simulink model "tiltrotor_model5"  (R2023a)
settings: Solver=FixedStepAuto  StartTime=0.0  StopTime=30  FixedStep=1e-3  RelTol=1e-3
values from neighbouring files (symbols this model uses):
  g = 9.81    [LQR_controller_pitching.m]    (also in MPC_controller_pitching.m; MPC_vs_LQR.m; simulation_parameters.m)
  I = diag([0.018 0.035 0.051])    [simulation_parameters.m]
  initial = [0 0 0 0 0 0]'    [simulation_parameters.m]
  kf = 65    [simulation_parameters.m]
  Lh = 0.2    [simulation_parameters.m]
  Lv = 0.2    [simulation_parameters.m]
  m = 1.12    [LQR_controller_pitching.m]    (also in MPC_vs_LQR.m = size(Bd,2); simulation_parameters.m)
  p_D = 0    [controller_parameters_model_5_and_6.m]
  p_I = 0    [controller_parameters_model_5_and_6.m]
  p_P = 0.35    [controller_parameters_model_5_and_6.m]
  pitch_D = 0.4    [controller_parameters.m]    (also in controller_parameters_model_3_and_4.m; controller_parameters_model_5_and_6.m = 0)
  pitch_I = 0    [controller_parameters.m]    (also in controller_parameters_model_3_and_4.m; controller_parameters_model_5_and_6.m)
  pitch_P = 1.4    [controller_parameters.m]    (also in controller_parameters_model_3_and_4.m; controller_parameters_model_5_and_6.m = 10)
  r_D = 0    [controller_parameters_model_5_and_6.m]
  r_I = 0    [controller_parameters_model_5_and_6.m]
  r_P = 1    [controller_parameters_model_5_and_6.m]
  reference = [1 1 1 0 40 50]'    [simulation_parameters.m]
  roll_D = 0.3    [controller_parameters.m]    (also in controller_parameters_model_3_and_4.m; controller_parameters_model_5_and_6.m = 1)
  roll_I = 0    [controller_parameters.m]    (also in controller_parameters_model_3_and_4.m; controller_parameters_model_5_and_6.m)
  roll_P = 1.5    [controller_parameters.m]    (also in controller_parameters_model_3_and_4.m; controller_parameters_model_5_and_6.m = 8)
  s_r = [1 1 1 1 1 1]    [simulation_parameters.m]
  Tmax = 4    [simulation_parameters.m]
  toll = 1e-12    [simulation_parameters.m]
  vy_D = 0    [controller_parameters.m]    (also in controller_parameters_model_3_and_4.m; controller_parameters_model_5_and_6.m)
  vy_I = 0    [controller_parameters.m]    (also in controller_parameters_model_3_and_4.m; controller_parameters_model_5_and_6.m)
  vy_P = 5    [controller_parameters.m]    (also in controller_parameters_model_3_and_4.m; controller_parameters_model_5_and_6.m = 12)
  x_D = 0.7    [controller_parameters.m]    (also in controller_parameters_model_3_and_4.m; controller_parameters_model_5_and_6.m = 0)
  x_I = 0    [controller_parameters.m]    (also in controller_parameters_model_3_and_4.m; controller_parameters_model_5_and_6.m)
  x_P = 1.8    [controller_parameters.m]    (also in controller_parameters_model_3_and_4.m; controller_parameters_model_5_and_6.m = 1.5)
  y_D = 0.7    [controller_parameters.m]    (also in controller_parameters_model_3_and_4.m; controller_parameters_model_5_and_6.m = 0.3)
  y_I = 0    [controller_parameters.m]    (also in controller_parameters_model_3_and_4.m; controller_parameters_model_5_and_6.m)
  y_P = 1.8    [controller_parameters.m]    (also in controller_parameters_model_3_and_4.m; controller_parameters_model_5_and_6.m = 1.5)
  yaw_D = 0.5    [controller_parameters.m]    (also in controller_parameters_model_3_and_4.m = 0.3; controller_parameters_model_5_and_6.m = 0)
  yaw_I = 0    [controller_parameters.m]    (also in controller_parameters_model_3_and_4.m; controller_parameters_model_5_and_6.m)
  yaw_P = 1    [controller_parameters.m]    (also in controller_parameters_model_3_and_4.m; controller_parameters_model_5_and_6.m = 1.5)
  z_D = 0    [controller_parameters.m]    (also in controller_parameters_model_3_and_4.m; controller_parameters_model_5_and_6.m)
  z_I = 0    [controller_parameters.m]    (also in controller_parameters_model_3_and_4.m; controller_parameters_model_5_and_6.m)
  z_P = 3    [controller_parameters.m]    (also in controller_parameters_model_3_and_4.m; controller_parameters_model_5_and_6.m = 2.5)
undefined symbols (not defined in the file or in its folder): K
libraries: slpidlib x9, simulink x6, simulink_extras x1, matrix_library x1
(part 1 of 2)
settings Model: Creator=and20  LastModifiedBy=and20

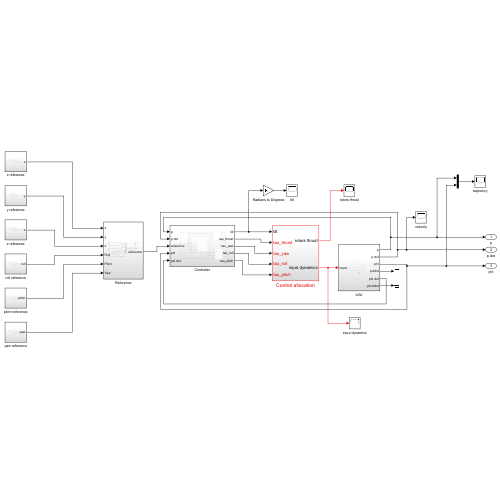
[thumbnail: Simulink's stored preview of the top-level diagram]
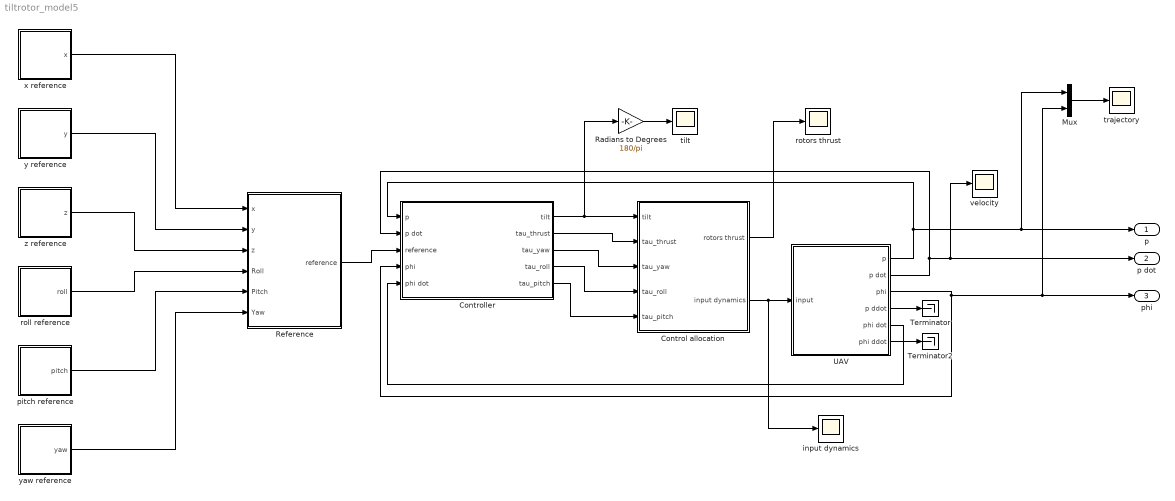
== system tiltrotor_model5 ==
  Control allocation : Subsystem
  Controller : Subsystem
  Mux : Mux  Inputs=2
  Radians to Degrees : Gain  Gain=180/pi
  Reference : Subsystem
  Terminator : Terminator
  Terminator2 : Terminator
  UAV : Subsystem
  input dynamics : Scope
  pitch reference : Subsystem
  roll reference : Subsystem
  rotors thrust : Scope
  tilt : Scope
  trajectory : Scope
  velocity : Scope
  x reference : Subsystem
  y reference : Subsystem
  yaw reference : Subsystem
  z reference : Subsystem
  p : Outport
  p dot : Outport  Port=2
  phi : Outport  Port=3
  wires:
  Reference/1(reference) -> Controller/3(reference)
  UAV/2(p dot) -> Controller/2(p dot), velocity/1, p dot/1
  UAV/3(phi) -> Mux/2, phi/1, Controller/4(phi)
  Mux/1 -> trajectory/1
  UAV/1(p) -> Controller/1(p), Mux/1, p/1
  x reference/1(x) -> Reference/1(x)
  y reference/1(y) -> Reference/2(y)
  z reference/1(z) -> Reference/3(z)
  roll reference/1(roll) -> Reference/4(Roll)
  pitch reference/1(pitch) -> Reference/5(Pitch)
  yaw reference/1(yaw) -> Reference/6(Yaw)
  Radians to Degrees/1 -> tilt/1
  UAV/4(p ddot) -> Terminator/1
  UAV/5(phi dot) -> Controller/5(phi dot)
  UAV/6(phi ddot) -> Terminator2/1
  Controller/1(tilt) -> Radians to Degrees/1, Control allocation/1(tilt)
  Controller/2(tau_thrust) -> Control allocation/2(tau_thrust)
  Controller/3(tau_yaw) -> Control allocation/3(tau_yaw)
  Controller/4(tau_roll) -> Control allocation/4(tau_roll)
  Controller/5(tau_pitch) -> Control allocation/5(tau_pitch)
  Control allocation/2(input dynamics) -> input dynamics/1, UAV/1(input)
  Control allocation/1(rotors thrust) -> rotors thrust/1

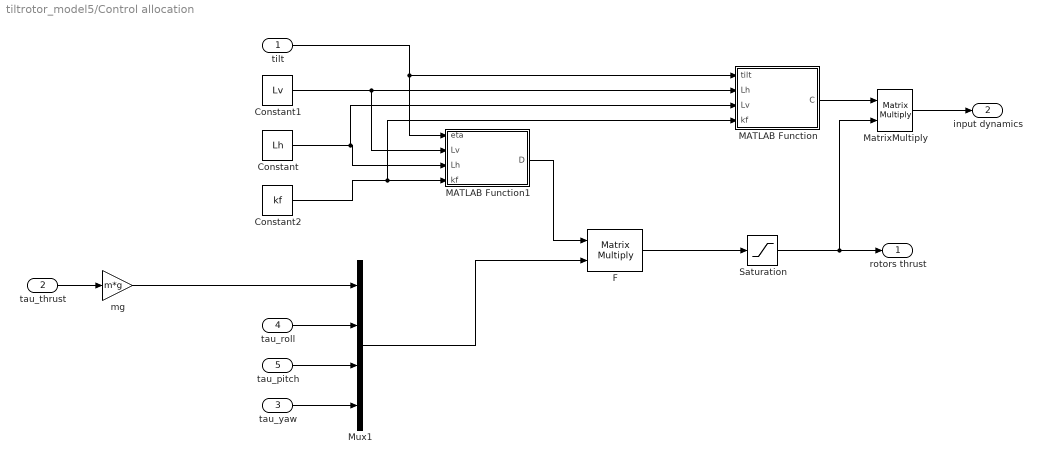
== system tiltrotor_model5/Control allocation ==
  tilt : Inport
  tau_thrust : Inport  Port=2
  tau_yaw : Inport  Port=3
  tau_roll : Inport  Port=4
  tau_pitch : Inport  Port=5
  Constant : Constant  Value=Lh
  Constant1 : Constant  Value=Lv
  Constant2 : Constant  Value=kf
  F : Product  Multiplication=Matrix(*)
  MATLAB Function : MATLAB Function  TreatAsAtomicUnit=on
  MATLAB Function1 : MATLAB Function  TreatAsAtomicUnit=on
  MatrixMultiply : Product  Multiplication=Matrix(*)
  Mux1 : Mux
  Saturation : Saturate  UpperLimit=Tmax  LowerLimit=0
  mg : Gain  Gain=m*g
  rotors thrust : Outport
  input dynamics : Outport  Port=2
  wires:
  MatrixMultiply/1 -> input dynamics/1
  tau_yaw/1 -> Mux1/4
  MATLAB Function1/1(D) -> F/1
  Constant1/1 -> MATLAB Function/2(Lh), MATLAB Function1/2(Lv)
  Constant2/1 -> MATLAB Function/4(kf), MATLAB Function1/4(kf)
  tau_roll/1 -> Mux1/2
  Mux1/1 -> F/2
  tau_thrust/1 -> mg/1
  tau_pitch/1 -> Mux1/3
  mg/1 -> Mux1/1
  tilt/1 -> MATLAB Function1/1(eta), MATLAB Function/1(tilt)
  Saturation/1 -> MatrixMultiply/2, rotors thrust/1
  MATLAB Function/1(C) -> MatrixMultiply/1
  Constant/1 -> MATLAB Function/3(Lv), MATLAB Function1/3(Lh)
  F/1 -> Saturation/1

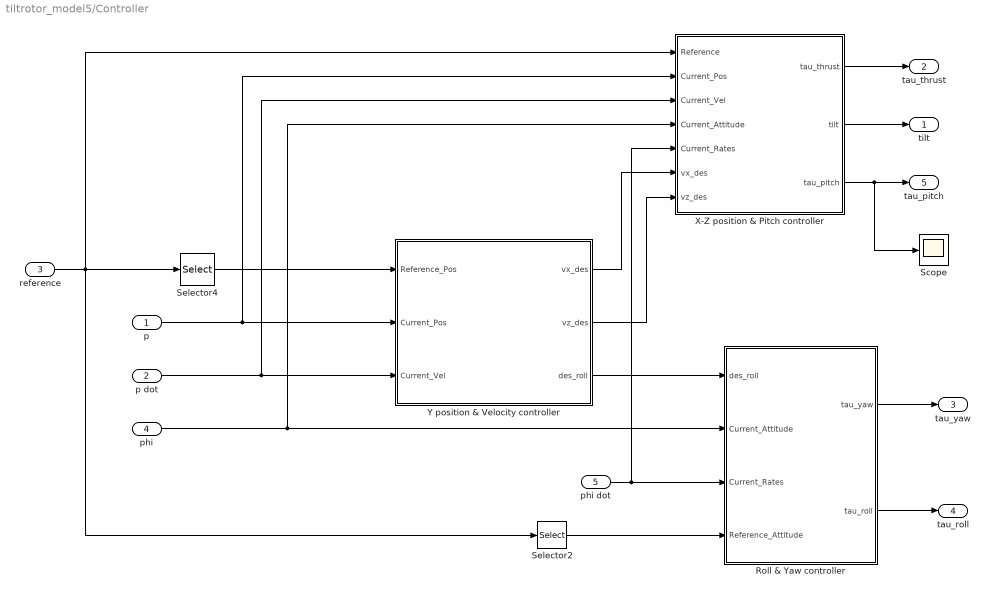
== system tiltrotor_model5/Controller ==
  p : Inport
  p dot : Inport  Port=2
  reference : Inport  Port=3
  phi : Inport  Port=4
  phi dot : Inport  Port=5
  Roll & Yaw controller : Subsystem
  Scope : Scope
  Selector2 : Selector  InputPortWidth=6  IndexOptions=Index vector (dialog)  Indices=[4 5]  OutputSizes=1
  Selector4 : Selector  InputPortWidth=6  IndexOptions=Index vector (dialog)  Indices=[1:3]  OutputSizes=1
  X-Z position & Pitch controller : Subsystem
  Y position & Velocity controller : Subsystem
  tilt : Outport
  tau_thrust : Outport  Port=2
  tau_yaw : Outport  Port=3
  tau_roll : Outport  Port=4
  tau_pitch : Outport  Port=5
  wires:
  reference/1 -> X-Z position & Pitch controller/1(Reference), Selector4/1, Selector2/1
  phi/1 -> X-Z position & Pitch controller/4(Current_Attitude), Roll & Yaw controller/2(Current_Attitude)
  Roll & Yaw controller/1(tau_yaw) -> tau_yaw/1
  Roll & Yaw controller/2(tau_roll) -> tau_roll/1
  Selector2/1 -> Roll & Yaw controller/4(Reference_Attitude)
  X-Z position & Pitch controller/3(tau_pitch) -> Scope/1, tau_pitch/1
  X-Z position & Pitch controller/2(tilt) -> tilt/1
  Selector4/1 -> Y position & Velocity controller/1(Reference_Pos)
  Y position & Velocity controller/3(des_roll) -> Roll & Yaw controller/1(des_roll)
  Y position & Velocity controller/1(vx_des) -> X-Z position & Pitch controller/6(vx_des)
  Y position & Velocity controller/2(vz_des) -> X-Z position & Pitch controller/7(vz_des)
  X-Z position & Pitch controller/1(tau_thrust) -> tau_thrust/1
  p/1 -> X-Z position & Pitch controller/2(Current_Pos), Y position & Velocity controller/2(Current_Pos)
  p dot/1 -> X-Z position & Pitch controller/3(Current_Vel), Y position & Velocity controller/3(Current_Vel)
  phi dot/1 -> X-Z position & Pitch controller/5(Current_Rates), Roll & Yaw controller/3(Current_Rates)

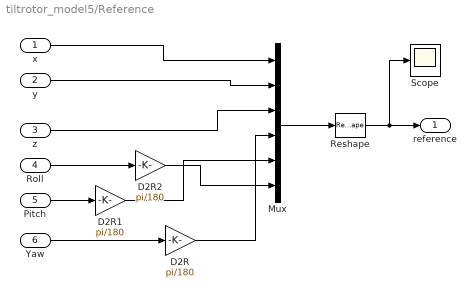
== system tiltrotor_model5/Reference ==
  x : Inport
  y : Inport  Port=2
  z : Inport  Port=3
  Roll : Inport  Port=4
  Pitch : Inport  Port=5
  Yaw : Inport  Port=6
  D2R : Gain  Gain=pi/180
  D2R1 : Gain  Gain=pi/180
  D2R2 : Gain  Gain=pi/180
  Mux : Mux  Inputs=6
  Reshape : Reshape
  Scope : Scope
  reference : Outport
  wires:
  Mux/1 -> Reshape/1
  y/1 -> Mux/2
  z/1 -> Mux/3
  x/1 -> Mux/1
  Reshape/1 -> Scope/1, reference/1
  Pitch/1 -> D2R1/1
  Yaw/1 -> D2R/1
  Roll/1 -> D2R2/1
  D2R1/1 -> Mux/5
  D2R2/1 -> Mux/6
  D2R/1 -> Mux/4

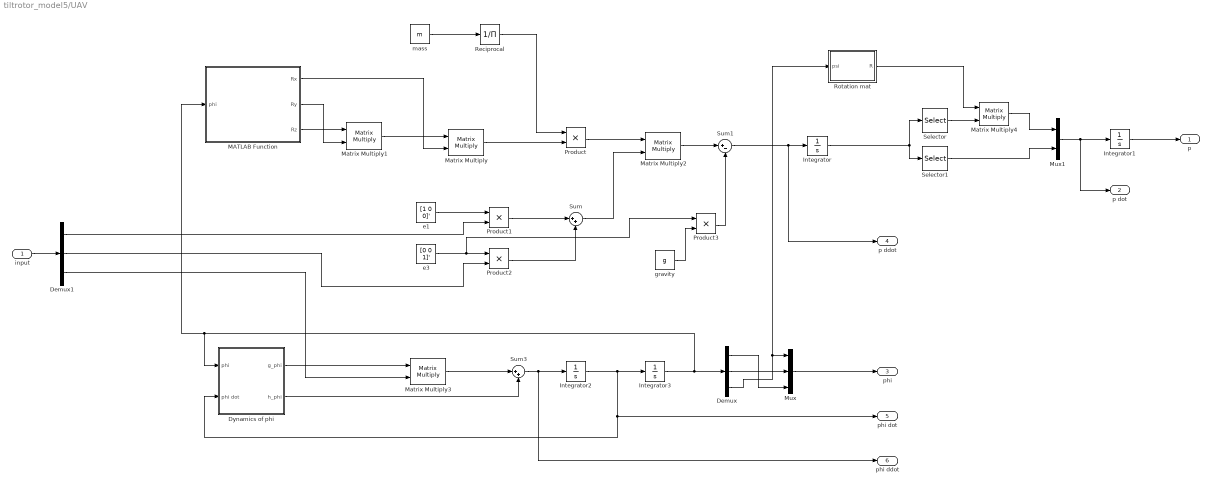
== system tiltrotor_model5/UAV ==
  input : Inport
  Demux : Demux  Outputs=3
  Demux1 : Demux  Outputs=[1 1 3]
  Dynamics of phi : Subsystem
  Integrator : Integrator  InitialCondition=zeros(3,1)
  Integrator1 : Integrator  InitialCondition=initial(1:3)
  Integrator2 : Integrator  InitialCondition=zeros(3,1)
  Integrator3 : Integrator  InitialCondition=initial(4:6)
  MATLAB Function : MATLAB Function  TreatAsAtomicUnit=on
  Matrix Multiply{,1..4} (5 alike) : Product  Multiplication=Matrix(*)
  Mux : Mux  Inputs=3
  Mux1 : Mux  Inputs=2
  Product{,1..3} (4 alike) : Product
  Reciprocal : Product  Inputs=/
  "Rotation mat " : MATLAB Function  TreatAsAtomicUnit=on
  Selector : Selector  InputPortWidth=3  IndexOptions=Index vector (dialog)  Indices=[1 2]  OutputSizes=1
  Selector1 : Selector  InputPortWidth=3  IndexOptions=Index vector (dialog)  Indices=[3]  OutputSizes=1
  Sum : Sum  Inputs=|++
  Sum1 : Sum  Inputs=|+-
  Sum3 : Sum  Inputs=|++
  e1 : Constant  Value=[1 0 0]'  VectorParams1D=off
  e3 : Constant  Value=[0 0 1]'  VectorParams1D=off
  gravity : Constant  Value=g
  mass : Constant  Value=m
  p : Outport
  p dot : Outport  Port=2
  phi : Outport  Port=3
  p ddot : Outport  Port=4
  phi dot : Outport  Port=5
  phi ddot : Outport  Port=6
  wires:
  Integrator2/1 -> Integrator3/1, phi dot/1, Dynamics of phi/2(phi dot)
  e3/1 -> Product3/1, Product2/1
  Matrix Multiply3/1 -> Sum3/1
  Product1/1 -> Sum/1
  MATLAB Function/1(Rx) -> Matrix Multiply/2
  Sum3/1 -> phi ddot/1, Integrator2/1
  Reciprocal/1 -> Product/1
  Integrator3/1 -> Demux/1, Dynamics of phi/1(phi), MATLAB Function/1(phi)
  Matrix Multiply2/1 -> Sum1/1
  mass/1 -> Reciprocal/1
  Product3/1 -> Sum1/2
  Dynamics of phi/1(g_phi) -> Matrix Multiply3/1
  Sum1/1 -> p ddot/1, Integrator/1
  Demux1/2 -> Product2/2
  e1/1 -> Product1/1
  Product/1 -> Matrix Multiply2/1
  Sum/1 -> Matrix Multiply2/2
  Demux1/1 -> Product1/2
  Matrix Multiply/1 -> Product/2
  Product2/1 -> Sum/2
  Dynamics of phi/2(h_phi) -> Sum3/2
  gravity/1 -> Product3/2
  Mux/1 -> phi/1
  Demux/2 -> Mux/2
  Demux/3 -> "Rotation mat "/1(psi), Mux/1
  Demux/1 -> Mux/3
  input/1 -> Demux1/1
  Demux1/3 -> Matrix Multiply3/2
  Matrix Multiply1/1 -> Matrix Multiply/1
  MATLAB Function/3(Rz) -> Matrix Multiply1/1
  MATLAB Function/2(Ry) -> Matrix Multiply1/2
  Integrator/1 -> Selector1/1, Selector/1
  Selector/1 -> Matrix Multiply4/2
  "Rotation mat "/1(R) -> Matrix Multiply4/1
  Matrix Multiply4/1 -> Mux1/1
  Mux1/1 -> p dot/1, Integrator1/1
  Selector1/1 -> Mux1/2
  Integrator1/1 -> p/1

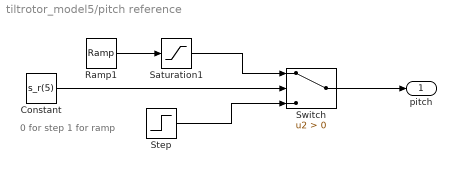
== system tiltrotor_model5/pitch reference ==
  note: 0 for step
      | 1 for ramp
  Constant : Constant  Value=s_r(5)
  Ramp1 : simulink/Sources/Ramp  slope=180/pi/4  start=25  InitialOutput=0
  Saturation1 : Saturate  UpperLimit=abs(reference(5))  LowerLimit=-abs(reference(5))
  Step : Step  Time=10  After=reference(5)  SampleTime=0
  Switch : Switch  Criteria=u2 > Threshold  SaturateOnIntegerOverflow=off  InputSameDT=off
  pitch : Outport
  wires:
  Ramp1/1 -> Saturation1/1
  Saturation1/1 -> Switch/1
  Switch/1 -> pitch/1
  Constant/1 -> Switch/2
  Step/1 -> Switch/3

== system tiltrotor_model5/roll reference ==
  note: 0 for step
      | 1 for ramp
  Constant1 : Constant  Value=s_r(4)
  Ramp2 : simulink/Sources/Ramp  slope=180/pi  start=10  InitialOutput=0
  Saturation2 : Saturate  UpperLimit=abs(reference(4))  LowerLimit=-abs(reference(4))
  Step : Step  Time=10  After=reference(4)  SampleTime=0
  Switch1 : Switch  Criteria=u2 > Threshold  SaturateOnIntegerOverflow=off  InputSameDT=off
  roll : Outport
  wires:
  Step/1 -> Switch1/3
  Ramp2/1 -> Saturation2/1
  Constant1/1 -> Switch1/2
  Saturation2/1 -> Switch1/1
  Switch1/1 -> roll/1

== system tiltrotor_model5/x reference ==
  note: 0 for step
      | 1 for ramp
  Constant : Constant  Value=s_r(1)
  Ramp1 : simulink/Sources/Ramp  slope=1  start=15  InitialOutput=0
  Saturation1 : Saturate  UpperLimit=abs(reference(1))  LowerLimit=-abs(reference(1))
  Step : Step  Time=10  After=reference(1)  SampleTime=0
  Switch : Switch  Criteria=u2 > Threshold  SaturateOnIntegerOverflow=off  InputSameDT=off
  x : Outport
  wires:
  Ramp1/1 -> Saturation1/1
  Saturation1/1 -> Switch/1
  Switch/1 -> x/1
  Constant/1 -> Switch/2
  Step/1 -> Switch/3

== system tiltrotor_model5/y reference ==
  note: 0 for step
      | 1 for ramp
  Constant1 : Constant  Value=s_r(2)
  Ramp2 : simulink/Sources/Ramp  slope=1  start=20  InitialOutput=0
  Saturation2 : Saturate  UpperLimit=abs(reference(2))  LowerLimit=-abs(reference(2))
  Step : Step  Time=10  After=reference(2)  SampleTime=0
  Switch1 : Switch  Criteria=u2 > Threshold  SaturateOnIntegerOverflow=off  InputSameDT=off
  y : Outport
  wires:
  Step/1 -> Switch1/3
  Ramp2/1 -> Saturation2/1
  Constant1/1 -> Switch1/2
  Saturation2/1 -> Switch1/1
  Switch1/1 -> y/1

== system tiltrotor_model5/yaw reference ==
  note: 0 for step
      | 1 for ramp
  Constant1 : Constant  Value=s_r(6)
  Ramp2 : simulink/Sources/Ramp  slope=180/pi/2  start=10  InitialOutput=0
  Saturation2 : Saturate  UpperLimit=abs(reference(6))  LowerLimit=-abs(reference(6))
  Step : Step  Time=10  After=reference(6)  SampleTime=0
  Switch1 : Switch  Criteria=u2 > Threshold  SaturateOnIntegerOverflow=off  InputSameDT=off
  yaw : Outport
  wires:
  Step/1 -> Switch1/3
  Ramp2/1 -> Saturation2/1
  Constant1/1 -> Switch1/2
  Saturation2/1 -> Switch1/1
  Switch1/1 -> yaw/1

== system tiltrotor_model5/z reference ==
  note: 0 for step
      | 1 for ramp
  Constant : Constant  Value=s_r(3)
  Ramp1 : simulink/Sources/Ramp  slope=1  start=5  InitialOutput=0
  Saturation1 : Saturate  UpperLimit=abs(reference(3))  LowerLimit=-abs(reference(3))
  Step : Step  Time=10  After=reference(3)  SampleTime=0
  Switch : Switch  Criteria=u2 > Threshold  SaturateOnIntegerOverflow=off  InputSameDT=off
  z : Outport
  wires:
  Ramp1/1 -> Saturation1/1
  Step/1 -> Switch/3
  Saturation1/1 -> Switch/1
  Switch/1 -> z/1
  Constant/1 -> Switch/2

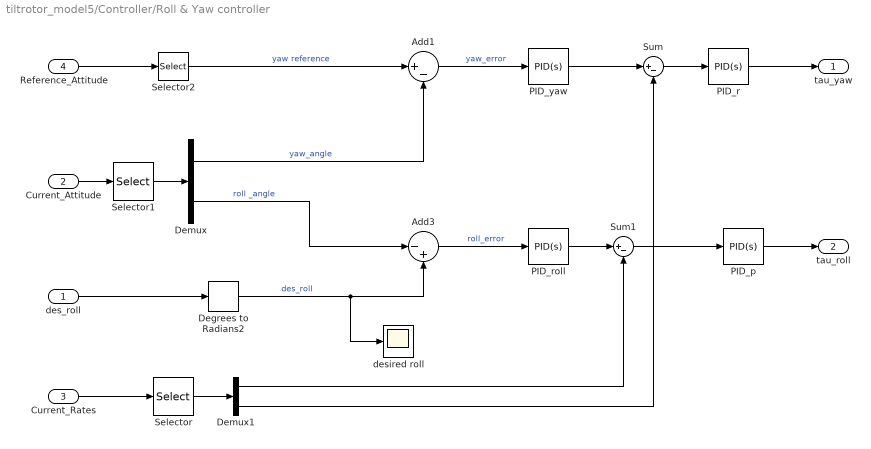
== system tiltrotor_model5/Controller/Roll & Yaw controller ==
  des_roll : Inport
  Current_Attitude : Inport  Port=2
  Current_Rates : Inport  Port=3
  Reference_Attitude : Inport  Port=4
  Add1 : Sum  Inputs=|+-
  Add3 : Sum  Inputs=|-+
  Degrees to Radians2 : simulink_extras/Transformations/Degrees to Radians
  Demux : Demux  Outputs=2
  Demux1 : Demux  Outputs=2
  PID_p : slpidlib/PID Controller  Controller=PID  Form=Parallel  TimeDomain=Continuous-time  UseExternalTs=off  SampleTime=-1  IntegratorMethod=Forward Euler  FilterMethod=Forward Euler  ControllerParametersSource=internal  P=p_P  I=p_I  UseKiTs=off  D=p_D  N=100  UseFilter=on  TunerSelectOption=Transfer Function Based (PID Tuner App)  InitialConditionSource=internal  InitialConditionForIntegrator=0  InitialConditionForFilter=0  DifferentiatorICPrevScaledInput=0  ExternalReset=none  TrackingMode=off  Kt=1  LimitOutput=off  SatLimitsSource=internal  UpperSaturationLimit=inf  LowerSaturationLimit=-inf  LinearizeAsGain=on  AntiWindupMode=none  Kb=1  LimitIntegrator=off  UpperIntegratorSaturationLimit=inf  LowerIntegratorSaturationLimit=-inf  POutMin=[]  POutMax=[]  IOutMin=[]  IOutMax=[]  DOutMin=[]  DOutMax=[]  NOutMin=[]  NOutMax=[]  SumOutMin=[]  SumOutMax=[]  SaturationOutMin=[]  SaturationOutMax=[]  PParamMin=[]  PParamMax=[]  IParamMin=[]  IParamMax=[]  DParamMin=[]  DParamMax=[]  NParamMin=[]  NParamMax=[]  KbParamMin=[]  KbParamMax=[]  KtParamMin=[]  KtParamMax=[]  KbOutMin=[]  KbOutMax=[]  KtOutMin=[]  KtOutMax=[]  IntegratorOutMin=[]  IntegratorOutMax=[]  FilterOutMin=[]  FilterOutMax=[]  SumI1OutMin=[]  SumI1OutMax=[]  SumI2OutMin=[]  SumI2OutMax=[]  SumI3OutMin=[]  SumI3OutMax=[]  SumI4OutMin=[]  SumI4OutMax=[]  SumDOutMin=[]  SumDOutMax=[]  DifferentiatorOutMin=[]  DifferentiatorOutMax=[]  FilterDiffOutCoefMin=[]  FilterDiffOutCoefMax=[]  ReciprocalOutMin=[]  ReciprocalOutMax=[]  SumDenOutMin=[]  SumDenOutMax=[]  SumNumOutMin=[]  SumNumOutMax=[]  DivideOutMin=[]  DivideOutMax=[]  UdiffTsProdOutMin=[]  UdiffTsProdOutMax=[]  NTsProdOutMin=[]  NTsProdOutMax=[]  UintegralTsProdOutMin=[]  UintegralTsProdOutMax=[]  UngainTsProdOutMin=[]  UngainTsProdOutMax=[]  ClampingZeroOutDataTypeStr=Inherit: Inherit via back propagation  ClampingZeroOutMin=[]  ClampingZeroOutMax=[]  FilterDenConstantOutDataTypeStr=Inherit: Inherit via back propagation  FilterDenConstantOutMin=[]  FilterDenConstantOutMax=[]  PCopyOutDataTypeStr=Inherit: Inherit via back propagation  PCopyOutMin=[]  PCopyOutMax=[]  NCopyOutDataTypeStr=Inherit: Inherit via back propagation  NCopyOutMin=[]  NCopyOutMax=[]  IntegratorContinuousStateAttributes=''  IntegratorStateMustResolveToSignalObject=off  IntegratorRTWStateStorageClass=Auto  FilterContinuousStateAttributes=''  FilterStateMustResolveToSignalObject=off  FilterRTWStateStorageClass=Auto  ParallelPVariant=InternalParameters  IdealPVariant=Disabled  IVariant=InternalParameters  DVariant=InternalParameters  IntegratorVariant=Continuous  SatVariant=Disabled  AWVariant=Passthrough  PCopyVariant=Disabled  TRVariant=Disabled  FdbkBlocksVariant=Forward  IdealPFdbkVariant=Disabled  SatFdbkVariant=Disabled  DerivativeFilterVariant=ContFilter  NVariant=InternalParameters  NCopyVariant=Disabled  FilterICVariant=InternalICsFilter  IntegratorICVariant=InternalICs  ExternalResetVariant=Disabled  TRSumVariant=Passthrough  SumFdbkVariant=Disabled  SumVariant=Sum_PID  TsampFilterVariant=InternalTs  TsampNgainVariant=Passthrough  TsampIntegralVariant=Disabled_SignalSpec  ExternalSaturationOutDataTypeStr=Inherit: Same as second input
  PID_r : slpidlib/PID Controller  Controller=PID  Form=Parallel  TimeDomain=Continuous-time  UseExternalTs=off  SampleTime=-1  IntegratorMethod=Forward Euler  FilterMethod=Forward Euler  ControllerParametersSource=internal  P=r_P  I=r_I  UseKiTs=off  D=r_D  N=100  UseFilter=on  TunerSelectOption=Transfer Function Based (PID Tuner App)  InitialConditionSource=internal  InitialConditionForIntegrator=0  InitialConditionForFilter=0  DifferentiatorICPrevScaledInput=0  ExternalReset=none  TrackingMode=off  Kt=1  LimitOutput=off  SatLimitsSource=internal  UpperSaturationLimit=inf  LowerSaturationLimit=-inf  LinearizeAsGain=on  AntiWindupMode=none  Kb=1  LimitIntegrator=off  UpperIntegratorSaturationLimit=inf  LowerIntegratorSaturationLimit=-inf  POutMin=[]  POutMax=[]  IOutMin=[]  IOutMax=[]  DOutMin=[]  DOutMax=[]  NOutMin=[]  NOutMax=[]  SumOutMin=[]  SumOutMax=[]  SaturationOutMin=[]  SaturationOutMax=[]  PParamMin=[]  PParamMax=[]  IParamMin=[]  IParamMax=[]  DParamMin=[]  DParamMax=[]  NParamMin=[]  NParamMax=[]  KbParamMin=[]  KbParamMax=[]  KtParamMin=[]  KtParamMax=[]  KbOutMin=[]  KbOutMax=[]  KtOutMin=[]  KtOutMax=[]  IntegratorOutMin=[]  IntegratorOutMax=[]  FilterOutMin=[]  FilterOutMax=[]  SumI1OutMin=[]  SumI1OutMax=[]  SumI2OutMin=[]  SumI2OutMax=[]  SumI3OutMin=[]  SumI3OutMax=[]  SumI4OutMin=[]  SumI4OutMax=[]  SumDOutMin=[]  SumDOutMax=[]  DifferentiatorOutMin=[]  DifferentiatorOutMax=[]  FilterDiffOutCoefMin=[]  FilterDiffOutCoefMax=[]  ReciprocalOutMin=[]  ReciprocalOutMax=[]  SumDenOutMin=[]  SumDenOutMax=[]  SumNumOutMin=[]  SumNumOutMax=[]  DivideOutMin=[]  DivideOutMax=[]  UdiffTsProdOutMin=[]  UdiffTsProdOutMax=[]  NTsProdOutMin=[]  NTsProdOutMax=[]  UintegralTsProdOutMin=[]  UintegralTsProdOutMax=[]  UngainTsProdOutMin=[]  UngainTsProdOutMax=[]  ClampingZeroOutDataTypeStr=Inherit: Inherit via back propagation  ClampingZeroOutMin=[]  ClampingZeroOutMax=[]  FilterDenConstantOutDataTypeStr=Inherit: Inherit via back propagation  FilterDenConstantOutMin=[]  FilterDenConstantOutMax=[]  PCopyOutDataTypeStr=Inherit: Inherit via back propagation  PCopyOutMin=[]  PCopyOutMax=[]  NCopyOutDataTypeStr=Inherit: Inherit via back propagation  NCopyOutMin=[]  NCopyOutMax=[]  IntegratorContinuousStateAttributes=''  IntegratorStateMustResolveToSignalObject=off  IntegratorRTWStateStorageClass=Auto  FilterContinuousStateAttributes=''  FilterStateMustResolveToSignalObject=off  FilterRTWStateStorageClass=Auto  ParallelPVariant=InternalParameters  IdealPVariant=Disabled  IVariant=InternalParameters  DVariant=InternalParameters  IntegratorVariant=Continuous  SatVariant=Disabled  AWVariant=Passthrough  PCopyVariant=Disabled  TRVariant=Disabled  FdbkBlocksVariant=Forward  IdealPFdbkVariant=Disabled  SatFdbkVariant=Disabled  DerivativeFilterVariant=ContFilter  NVariant=InternalParameters  NCopyVariant=Disabled  FilterICVariant=InternalICsFilter  IntegratorICVariant=InternalICs  ExternalResetVariant=Disabled  TRSumVariant=Passthrough  SumFdbkVariant=Disabled  SumVariant=Sum_PID  TsampFilterVariant=InternalTs  TsampNgainVariant=Passthrough  TsampIntegralVariant=Disabled_SignalSpec  ExternalSaturationOutDataTypeStr=Inherit: Same as second input
  PID_roll : slpidlib/PID Controller  Controller=PID  Form=Parallel  TimeDomain=Continuous-time  UseExternalTs=off  SampleTime=-1  IntegratorMethod=Backward Euler  FilterMethod=Forward Euler  ControllerParametersSource=internal  P=roll_P  I=roll_I  UseKiTs=off  D=roll_D  N=100  UseFilter=on  TunerSelectOption=Transfer Function Based (PID Tuner App)  InitialConditionSource=internal  InitialConditionForIntegrator=0  InitialConditionForFilter=0  DifferentiatorICPrevScaledInput=0  ExternalReset=none  TrackingMode=off  Kt=1  LimitOutput=off  SatLimitsSource=internal  UpperSaturationLimit=0.05  LowerSaturationLimit=-0.05  LinearizeAsGain=off  AntiWindupMode=none  Kb=1  LimitIntegrator=off  UpperIntegratorSaturationLimit=inf  LowerIntegratorSaturationLimit=-inf  POutMin=[]  POutMax=[]  IOutMin=[]  IOutMax=[]  DOutMin=[]  DOutMax=[]  NOutMin=[]  NOutMax=[]  SumOutMin=[]  SumOutMax=[]  SaturationOutMin=[]  SaturationOutMax=[]  PParamMin=[]  PParamMax=[]  IParamMin=[]  IParamMax=[]  DParamMin=[]  DParamMax=[]  NParamMin=[]  NParamMax=[]  KbParamMin=[]  KbParamMax=[]  KtParamMin=[]  KtParamMax=[]  KbOutMin=[]  KbOutMax=[]  KtOutMin=[]  KtOutMax=[]  IntegratorOutMin=[]  IntegratorOutMax=[]  FilterOutMin=[]  FilterOutMax=[]  SumI1OutMin=[]  SumI1OutMax=[]  SumI2OutMin=[]  SumI2OutMax=[]  SumI3OutMin=[]  SumI3OutMax=[]  SumI4OutMin=[]  SumI4OutMax=[]  SumDOutMin=[]  SumDOutMax=[]  DifferentiatorOutMin=[]  DifferentiatorOutMax=[]  FilterDiffOutCoefMin=[]  FilterDiffOutCoefMax=[]  ReciprocalOutMin=[]  ReciprocalOutMax=[]  SumDenOutMin=[]  SumDenOutMax=[]  SumNumOutMin=[]  SumNumOutMax=[]  DivideOutMin=[]  DivideOutMax=[]  UdiffTsProdOutMin=[]  UdiffTsProdOutMax=[]  NTsProdOutMin=[]  NTsProdOutMax=[]  UintegralTsProdOutMin=[]  UintegralTsProdOutMax=[]  UngainTsProdOutMin=[]  UngainTsProdOutMax=[]  ClampingZeroOutDataTypeStr=Inherit: Inherit via back propagation  ClampingZeroOutMin=[]  ClampingZeroOutMax=[]  FilterDenConstantOutDataTypeStr=Inherit: Inherit via back propagation  FilterDenConstantOutMin=[]  FilterDenConstantOutMax=[]  PCopyOutDataTypeStr=Inherit: Inherit via back propagation  PCopyOutMin=[]  PCopyOutMax=[]  NCopyOutDataTypeStr=Inherit: Inherit via back propagation  NCopyOutMin=[]  NCopyOutMax=[]  IntegratorContinuousStateAttributes=''  IntegratorStateMustResolveToSignalObject=off  IntegratorRTWStateStorageClass=Auto  FilterContinuousStateAttributes=''  FilterStateMustResolveToSignalObject=off  FilterRTWStateStorageClass=Auto  ParallelPVariant=InternalParameters  IdealPVariant=Disabled  IVariant=InternalParameters  DVariant=InternalParameters  IntegratorVariant=Continuous  SatVariant=Disabled  AWVariant=Passthrough  PCopyVariant=Disabled  TRVariant=Disabled  FdbkBlocksVariant=Forward  IdealPFdbkVariant=Disabled  SatFdbkVariant=Disabled  DerivativeFilterVariant=ContFilter  NVariant=InternalParameters  NCopyVariant=Disabled  FilterICVariant=InternalICsFilter  IntegratorICVariant=InternalICs  ExternalResetVariant=Disabled  TRSumVariant=Passthrough  SumFdbkVariant=Disabled  SumVariant=Sum_PID  TsampFilterVariant=InternalTs  TsampNgainVariant=Passthrough  TsampIntegralVariant=Disabled_SignalSpec  ExternalSaturationOutDataTypeStr=Inherit: Same as second input
  PID_yaw : slpidlib/PID Controller  Controller=PID  Form=Parallel  TimeDomain=Continuous-time  UseExternalTs=off  SampleTime=-1  IntegratorMethod=Backward Euler  FilterMethod=Forward Euler  ControllerParametersSource=internal  P=yaw_P  I=yaw_I  UseKiTs=off  D=yaw_D  N=100  UseFilter=on  TunerSelectOption=Transfer Function Based (PID Tuner App)  InitialConditionSource=internal  InitialConditionForIntegrator=0  InitialConditionForFilter=0  DifferentiatorICPrevScaledInput=0  ExternalReset=none  TrackingMode=off  Kt=1  LimitOutput=off  SatLimitsSource=internal  UpperSaturationLimit=0.01  LowerSaturationLimit=-0.01  LinearizeAsGain=off  AntiWindupMode=clamping  Kb=1  LimitIntegrator=off  UpperIntegratorSaturationLimit=inf  LowerIntegratorSaturationLimit=-inf  POutMin=[]  POutMax=[]  IOutMin=[]  IOutMax=[]  DOutMin=[]  DOutMax=[]  NOutMin=[]  NOutMax=[]  SumOutMin=[]  SumOutMax=[]  SaturationOutMin=[]  SaturationOutMax=[]  PParamMin=[]  PParamMax=[]  IParamMin=[]  IParamMax=[]  DParamMin=[]  DParamMax=[]  NParamMin=[]  NParamMax=[]  KbParamMin=[]  KbParamMax=[]  KtParamMin=[]  KtParamMax=[]  KbOutMin=[]  KbOutMax=[]  KtOutMin=[]  KtOutMax=[]  IntegratorOutMin=[]  IntegratorOutMax=[]  FilterOutMin=[]  FilterOutMax=[]  SumI1OutMin=[]  SumI1OutMax=[]  SumI2OutMin=[]  SumI2OutMax=[]  SumI3OutMin=[]  SumI3OutMax=[]  SumI4OutMin=[]  SumI4OutMax=[]  SumDOutMin=[]  SumDOutMax=[]  DifferentiatorOutMin=[]  DifferentiatorOutMax=[]  FilterDiffOutCoefMin=[]  FilterDiffOutCoefMax=[]  ReciprocalOutMin=[]  ReciprocalOutMax=[]  SumDenOutMin=[]  SumDenOutMax=[]  SumNumOutMin=[]  SumNumOutMax=[]  DivideOutMin=[]  DivideOutMax=[]  UdiffTsProdOutMin=[]  UdiffTsProdOutMax=[]  NTsProdOutMin=[]  NTsProdOutMax=[]  UintegralTsProdOutMin=[]  UintegralTsProdOutMax=[]  UngainTsProdOutMin=[]  UngainTsProdOutMax=[]  ClampingZeroOutDataTypeStr=Inherit: Inherit via back propagation  ClampingZeroOutMin=[]  ClampingZeroOutMax=[]  FilterDenConstantOutDataTypeStr=Inherit: Inherit via back propagation  FilterDenConstantOutMin=[]  FilterDenConstantOutMax=[]  PCopyOutDataTypeStr=Inherit: Inherit via back propagation  PCopyOutMin=[]  PCopyOutMax=[]  NCopyOutDataTypeStr=Inherit: Inherit via back propagation  NCopyOutMin=[]  NCopyOutMax=[]  IntegratorContinuousStateAttributes=''  IntegratorStateMustResolveToSignalObject=off  IntegratorRTWStateStorageClass=Auto  FilterContinuousStateAttributes=''  FilterStateMustResolveToSignalObject=off  FilterRTWStateStorageClass=Auto  ParallelPVariant=InternalParameters  IdealPVariant=Disabled  IVariant=InternalParameters  DVariant=InternalParameters  IntegratorVariant=Continuous  SatVariant=Disabled  AWVariant=Passthrough  PCopyVariant=Disabled  TRVariant=Disabled  FdbkBlocksVariant=Forward  IdealPFdbkVariant=Disabled  SatFdbkVariant=Disabled  DerivativeFilterVariant=ContFilter  NVariant=InternalParameters  NCopyVariant=Disabled  FilterICVariant=InternalICsFilter  IntegratorICVariant=InternalICs  ExternalResetVariant=Disabled  TRSumVariant=Passthrough  SumFdbkVariant=Disabled  SumVariant=Sum_PID  TsampFilterVariant=InternalTs  TsampNgainVariant=Passthrough  TsampIntegralVariant=Disabled_SignalSpec  ExternalSaturationOutDataTypeStr=Inherit: Same as second input
  Selector : Selector  InputPortWidth=3  IndexOptions=Index vector (dialog)  Indices=[1 3]  OutputSizes=1
  Selector1 : Selector  InputPortWidth=3  IndexOptions=Index vector (dialog)  Indices=[1 3]  OutputSizes=1
  Selector2 : Selector  InputPortWidth=2  IndexOptions=Index vector (dialog)  Indices=[1]  OutputSizes=1
  Sum : Sum  Inputs=|+-
  Sum1 : Sum  Inputs=|+-
  desired roll : Scope
  tau_yaw : Outport
  tau_roll : Outport  Port=2
  wires:
  Add3/1 -> PID_roll/1  "roll_error"
  Add1/1 -> PID_yaw/1  "yaw_error"
  des_roll/1 -> Degrees to Radians2/1
  Degrees to Radians2/1 -> Add3/2, desired roll/1  "des_roll"
  Reference_Attitude/1 -> Selector2/1
  Current_Attitude/1 -> Selector1/1
  Demux/1 -> Add1/2  "yaw_angle"
  PID_r/1 -> tau_yaw/1
  Sum/1 -> PID_r/1
  Sum1/1 -> PID_p/1
  PID_p/1 -> tau_roll/1
  Current_Rates/1 -> Selector/1
  Selector/1 -> Demux1/1
  Demux1/1 -> Sum1/2
  Demux1/2 -> Sum/2
  PID_roll/1 -> Sum1/1
  PID_yaw/1 -> Sum/1
  Demux/2 -> Add3/1  "roll _angle"
  Selector2/1 -> Add1/1  "yaw reference"
  Selector1/1 -> Demux/1

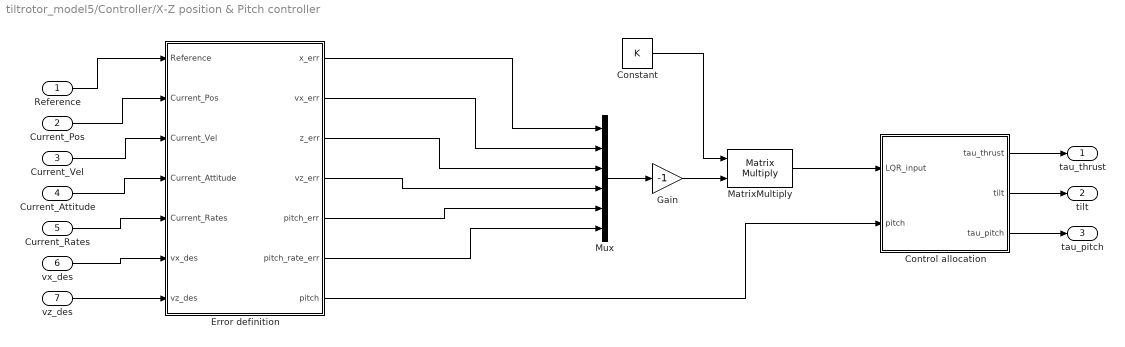
== system tiltrotor_model5/Controller/X-Z position & Pitch controller ==
  Reference : Inport
  Current_Pos : Inport  Port=2
  Current_Vel : Inport  Port=3
  Current_Attitude : Inport  Port=4
  Current_Rates : Inport  Port=5
  vx_des : Inport  Port=6
  vz_des : Inport  Port=7
  Constant : Constant  Value=K  VectorParams1D=off
  Control allocation : Subsystem
  Error definition : Subsystem
  Gain : Gain  Gain=-1
  MatrixMultiply : Product  Multiplication=Matrix(*)
  Mux : Mux  Inputs=6
  tau_thrust : Outport
  tilt : Outport  Port=2
  tau_pitch : Outport  Port=3
  wires:
  Gain/1 -> MatrixMultiply/2
  Mux/1 -> Gain/1
  Constant/1 -> MatrixMultiply/1
  MatrixMultiply/1 -> Control allocation/1(LQR_input)
  Control allocation/1(tau_thrust) -> tau_thrust/1
  Control allocation/2(tilt) -> tilt/1
  Control allocation/3(tau_pitch) -> tau_pitch/1
  Reference/1 -> Error definition/1(Reference)
  Current_Pos/1 -> Error definition/2(Current_Pos)
  Current_Vel/1 -> Error definition/3(Current_Vel)
  Current_Attitude/1 -> Error definition/4(Current_Attitude)
  Current_Rates/1 -> Error definition/5(Current_Rates)
  vx_des/1 -> Error definition/6(vx_des)
  vz_des/1 -> Error definition/7(vz_des)
  Error definition/1(x_err) -> Mux/1
  Error definition/2(vx_err) -> Mux/2
  Error definition/3(z_err) -> Mux/3
  Error definition/4(vz_err) -> Mux/4
  Error definition/7(pitch) -> Control allocation/2(pitch)
  Error definition/5(pitch_err) -> Mux/5
  Error definition/6(pitch_rate_err) -> Mux/6

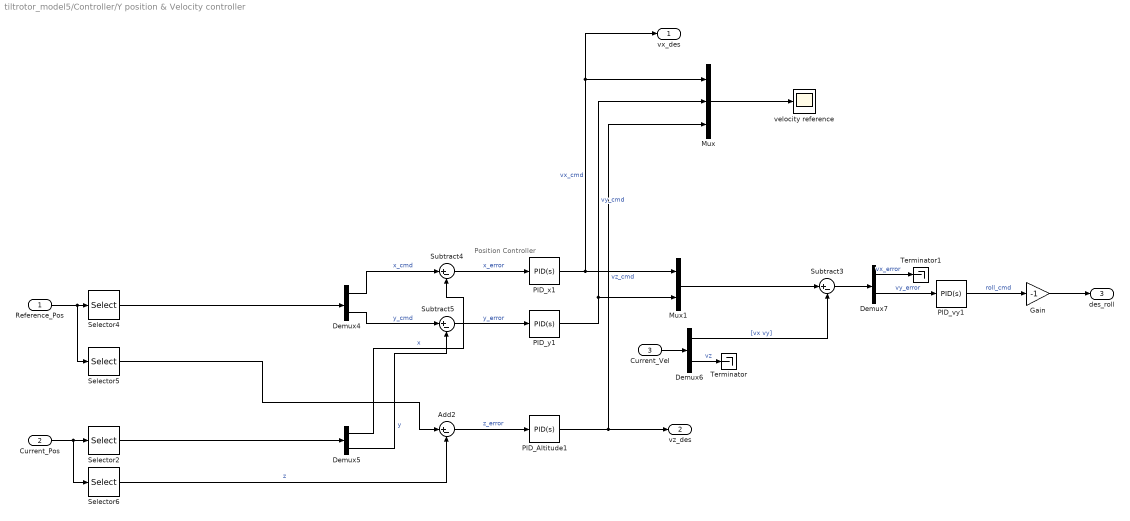
== system tiltrotor_model5/Controller/Y position & Velocity controller ==
  note: Position Controller
  Reference_Pos : Inport
  Current_Pos : Inport  Port=2
  Current_Vel : Inport  Port=3
  Add2 : Sum  Inputs=|+-
  Demux4 : Demux  Outputs=2
  Demux5 : Demux  Outputs=2
  Demux6 : Demux  Outputs=[2 1]
  Demux7 : Demux  Outputs=2
  Gain : Gain  Gain=-1
  Mux : Mux  Inputs=3
  Mux1 : Mux  Inputs=2
  PID_Altitude1 : slpidlib/PID Controller  Controller=PID  Form=Parallel  TimeDomain=Continuous-time  UseExternalTs=off  SampleTime=-1  IntegratorMethod=Backward Euler  FilterMethod=Forward Euler  ControllerParametersSource=internal  P=z_P  I=z_I  UseKiTs=off  D=z_D  N=100  UseFilter=on  TunerSelectOption=Transfer Function Based (PID Tuner App)  InitialConditionSource=internal  InitialConditionForIntegrator=0  InitialConditionForFilter=0  DifferentiatorICPrevScaledInput=0  ExternalReset=none  TrackingMode=off  Kt=1  LimitOutput=on  SatLimitsSource=internal  UpperSaturationLimit=10  LowerSaturationLimit=-10  LinearizeAsGain=off  AntiWindupMode=clamping  Kb=1  LimitIntegrator=off  UpperIntegratorSaturationLimit=inf  LowerIntegratorSaturationLimit=-inf  POutMin=[]  POutMax=[]  IOutMin=[]  IOutMax=[]  DOutMin=[]  DOutMax=[]  NOutMin=[]  NOutMax=[]  SumOutMin=[]  SumOutMax=[]  SaturationOutMin=[]  SaturationOutMax=[]  PParamMin=[]  PParamMax=[]  IParamMin=[]  IParamMax=[]  DParamMin=[]  DParamMax=[]  NParamMin=[]  NParamMax=[]  KbParamMin=[]  KbParamMax=[]  KtParamMin=[]  KtParamMax=[]  KbOutMin=[]  KbOutMax=[]  KtOutMin=[]  KtOutMax=[]  IntegratorOutMin=[]  IntegratorOutMax=[]  FilterOutMin=[]  FilterOutMax=[]  SumI1OutMin=[]  SumI1OutMax=[]  SumI2OutMin=[]  SumI2OutMax=[]  SumI3OutMin=[]  SumI3OutMax=[]  SumI4OutMin=[]  SumI4OutMax=[]  SumDOutMin=[]  SumDOutMax=[]  DifferentiatorOutMin=[]  DifferentiatorOutMax=[]  FilterDiffOutCoefMin=[]  FilterDiffOutCoefMax=[]  ReciprocalOutMin=[]  ReciprocalOutMax=[]  SumDenOutMin=[]  SumDenOutMax=[]  SumNumOutMin=[]  SumNumOutMax=[]  DivideOutMin=[]  DivideOutMax=[]  UdiffTsProdOutMin=[]  UdiffTsProdOutMax=[]  NTsProdOutMin=[]  NTsProdOutMax=[]  UintegralTsProdOutMin=[]  UintegralTsProdOutMax=[]  UngainTsProdOutMin=[]  UngainTsProdOutMax=[]  ClampingZeroOutDataTypeStr=Inherit: Inherit via back propagation  ClampingZeroOutMin=[]  ClampingZeroOutMax=[]  FilterDenConstantOutDataTypeStr=Inherit: Inherit via back propagation  FilterDenConstantOutMin=[]  FilterDenConstantOutMax=[]  PCopyOutDataTypeStr=Inherit: Inherit via back propagation  PCopyOutMin=[]  PCopyOutMax=[]  NCopyOutDataTypeStr=Inherit: Inherit via back propagation  NCopyOutMin=[]  NCopyOutMax=[]  IntegratorContinuousStateAttributes=''  IntegratorStateMustResolveToSignalObject=off  IntegratorRTWStateStorageClass=Auto  FilterContinuousStateAttributes=''  FilterStateMustResolveToSignalObject=off  FilterRTWStateStorageClass=Auto  ParallelPVariant=InternalParameters  IdealPVariant=Disabled  IVariant=InternalParameters  DVariant=InternalParameters  IntegratorVariant=Continuous  SatVariant=Enabled  AWVariant=ContClampingParallel  PCopyVariant=Disabled  TRVariant=Disabled  FdbkBlocksVariant=Forward  IdealPFdbkVariant=Disabled  SatFdbkVariant=Disabled  DerivativeFilterVariant=ContFilter  NVariant=InternalParameters  NCopyVariant=Disabled  FilterICVariant=InternalICsFilter  IntegratorICVariant=InternalICs  ExternalResetVariant=Disabled  TRSumVariant=Passthrough  SumFdbkVariant=Disabled  SumVariant=Sum_PID  TsampFilterVariant=InternalTs  TsampNgainVariant=Passthrough  TsampIntegralVariant=Disabled_SignalSpec  ExternalSaturationOutDataTypeStr=Inherit: Same as second input
  PID_vy1 : slpidlib/PID Controller  Controller=PID  Form=Parallel  TimeDomain=Continuous-time  UseExternalTs=off  SampleTime=-1  IntegratorMethod=Forward Euler  FilterMethod=Forward Euler  ControllerParametersSource=internal  P=vy_P  I=vy_I  UseKiTs=off  D=vy_D  N=100  UseFilter=on  TunerSelectOption=Frequency Response Based  InitialConditionSource=internal  InitialConditionForIntegrator=0  InitialConditionForFilter=0  DifferentiatorICPrevScaledInput=0  ExternalReset=none  TrackingMode=off  Kt=1  LimitOutput=on  SatLimitsSource=internal  UpperSaturationLimit=50  LowerSaturationLimit=-50  LinearizeAsGain=off  AntiWindupMode=none  Kb=1  LimitIntegrator=off  UpperIntegratorSaturationLimit=inf  LowerIntegratorSaturationLimit=-inf  POutMin=[]  POutMax=[]  IOutMin=[]  IOutMax=[]  DOutMin=[]  DOutMax=[]  NOutMin=[]  NOutMax=[]  SumOutMin=[]  SumOutMax=[]  SaturationOutMin=[]  SaturationOutMax=[]  PParamMin=[]  PParamMax=[]  IParamMin=[]  IParamMax=[]  DParamMin=[]  DParamMax=[]  NParamMin=[]  NParamMax=[]  KbParamMin=[]  KbParamMax=[]  KtParamMin=[]  KtParamMax=[]  KbOutMin=[]  KbOutMax=[]  KtOutMin=[]  KtOutMax=[]  IntegratorOutMin=[]  IntegratorOutMax=[]  FilterOutMin=[]  FilterOutMax=[]  SumI1OutMin=[]  SumI1OutMax=[]  SumI2OutMin=[]  SumI2OutMax=[]  SumI3OutMin=[]  SumI3OutMax=[]  SumI4OutMin=[]  SumI4OutMax=[]  SumDOutMin=[]  SumDOutMax=[]  DifferentiatorOutMin=[]  DifferentiatorOutMax=[]  FilterDiffOutCoefMin=[]  FilterDiffOutCoefMax=[]  ReciprocalOutMin=[]  ReciprocalOutMax=[]  SumDenOutMin=[]  SumDenOutMax=[]  SumNumOutMin=[]  SumNumOutMax=[]  DivideOutMin=[]  DivideOutMax=[]  UdiffTsProdOutMin=[]  UdiffTsProdOutMax=[]  NTsProdOutMin=[]  NTsProdOutMax=[]  UintegralTsProdOutMin=[]  UintegralTsProdOutMax=[]  UngainTsProdOutMin=[]  UngainTsProdOutMax=[]  ClampingZeroOutDataTypeStr=Inherit: Inherit via back propagation  ClampingZeroOutMin=[]  ClampingZeroOutMax=[]  FilterDenConstantOutDataTypeStr=Inherit: Inherit via back propagation  FilterDenConstantOutMin=[]  FilterDenConstantOutMax=[]  PCopyOutDataTypeStr=Inherit: Inherit via back propagation  PCopyOutMin=[]  PCopyOutMax=[]  NCopyOutDataTypeStr=Inherit: Inherit via back propagation  NCopyOutMin=[]  NCopyOutMax=[]  IntegratorContinuousStateAttributes=''  IntegratorStateMustResolveToSignalObject=off  IntegratorRTWStateStorageClass=Auto  FilterContinuousStateAttributes=''  FilterStateMustResolveToSignalObject=off  FilterRTWStateStorageClass=Auto  ParallelPVariant=InternalParameters  IdealPVariant=Disabled  IVariant=InternalParameters  DVariant=InternalParameters  IntegratorVariant=Continuous  SatVariant=Enabled  AWVariant=Passthrough  PCopyVariant=Disabled  TRVariant=Disabled  FdbkBlocksVariant=Forward  IdealPFdbkVariant=Disabled  SatFdbkVariant=Disabled  DerivativeFilterVariant=ContFilter  NVariant=InternalParameters  NCopyVariant=Disabled  FilterICVariant=InternalICsFilter  IntegratorICVariant=InternalICs  ExternalResetVariant=Disabled  TRSumVariant=Passthrough  SumFdbkVariant=Disabled  SumVariant=Sum_PID  TsampFilterVariant=InternalTs  TsampNgainVariant=Passthrough  TsampIntegralVariant=Disabled_SignalSpec  ExternalSaturationOutDataTypeStr=Inherit: Same as second input
  PID_x1 : slpidlib/PID Controller  Controller=PID  Form=Parallel  TimeDomain=Continuous-time  UseExternalTs=off  SampleTime=-1  IntegratorMethod=Forward Euler  FilterMethod=Forward Euler  ControllerParametersSource=internal  P=x_P  I=x_I  UseKiTs=off  D=x_D  N=100  UseFilter=on  TunerSelectOption=Frequency Response Based  InitialConditionSource=internal  InitialConditionForIntegrator=0  InitialConditionForFilter=0  DifferentiatorICPrevScaledInput=0  ExternalReset=none  TrackingMode=off  Kt=1  LimitOutput=on  SatLimitsSource=internal  UpperSaturationLimit=20  LowerSaturationLimit=-20  LinearizeAsGain=off  AntiWindupMode=clamping  Kb=1  LimitIntegrator=off  UpperIntegratorSaturationLimit=inf  LowerIntegratorSaturationLimit=-inf  POutMin=[]  POutMax=[]  IOutMin=[]  IOutMax=[]  DOutMin=[]  DOutMax=[]  NOutMin=[]  NOutMax=[]  SumOutMin=[]  SumOutMax=[]  SaturationOutMin=[]  SaturationOutMax=[]  PParamMin=[]  PParamMax=[]  IParamMin=[]  IParamMax=[]  DParamMin=[]  DParamMax=[]  NParamMin=[]  NParamMax=[]  KbParamMin=[]  KbParamMax=[]  KtParamMin=[]  KtParamMax=[]  KbOutMin=[]  KbOutMax=[]  KtOutMin=[]  KtOutMax=[]  IntegratorOutMin=[]  IntegratorOutMax=[]  FilterOutMin=[]  FilterOutMax=[]  SumI1OutMin=[]  SumI1OutMax=[]  SumI2OutMin=[]  SumI2OutMax=[]  SumI3OutMin=[]  SumI3OutMax=[]  SumI4OutMin=[]  SumI4OutMax=[]  SumDOutMin=[]  SumDOutMax=[]  DifferentiatorOutMin=[]  DifferentiatorOutMax=[]  FilterDiffOutCoefMin=[]  FilterDiffOutCoefMax=[]  ReciprocalOutMin=[]  ReciprocalOutMax=[]  SumDenOutMin=[]  SumDenOutMax=[]  SumNumOutMin=[]  SumNumOutMax=[]  DivideOutMin=[]  DivideOutMax=[]  UdiffTsProdOutMin=[]  UdiffTsProdOutMax=[]  NTsProdOutMin=[]  NTsProdOutMax=[]  UintegralTsProdOutMin=[]  UintegralTsProdOutMax=[]  UngainTsProdOutMin=[]  UngainTsProdOutMax=[]  ClampingZeroOutDataTypeStr=Inherit: Inherit via back propagation  ClampingZeroOutMin=[]  ClampingZeroOutMax=[]  FilterDenConstantOutDataTypeStr=Inherit: Inherit via back propagation  FilterDenConstantOutMin=[]  FilterDenConstantOutMax=[]  PCopyOutDataTypeStr=Inherit: Inherit via back propagation  PCopyOutMin=[]  PCopyOutMax=[]  NCopyOutDataTypeStr=Inherit: Inherit via back propagation  NCopyOutMin=[]  NCopyOutMax=[]  IntegratorContinuousStateAttributes=''  IntegratorStateMustResolveToSignalObject=off  IntegratorRTWStateStorageClass=Auto  FilterContinuousStateAttributes=''  FilterStateMustResolveToSignalObject=off  FilterRTWStateStorageClass=Auto  ParallelPVariant=InternalParameters  IdealPVariant=Disabled  IVariant=InternalParameters  DVariant=InternalParameters  IntegratorVariant=Continuous  SatVariant=Enabled  AWVariant=ContClampingParallel  PCopyVariant=Disabled  TRVariant=Disabled  FdbkBlocksVariant=Forward  IdealPFdbkVariant=Disabled  SatFdbkVariant=Disabled  DerivativeFilterVariant=ContFilter  NVariant=InternalParameters  NCopyVariant=Disabled  FilterICVariant=InternalICsFilter  IntegratorICVariant=InternalICs  ExternalResetVariant=Disabled  TRSumVariant=Passthrough  SumFdbkVariant=Disabled  SumVariant=Sum_PID  TsampFilterVariant=InternalTs  TsampNgainVariant=Passthrough  TsampIntegralVariant=Disabled_SignalSpec  ExternalSaturationOutDataTypeStr=Inherit: Same as second input
  PID_y1 : slpidlib/PID Controller  Controller=PID  Form=Parallel  TimeDomain=Continuous-time  UseExternalTs=off  SampleTime=-1  IntegratorMethod=Forward Euler  FilterMethod=Forward Euler  ControllerParametersSource=internal  P=y_P  I=y_I  UseKiTs=off  D=y_D  N=100  UseFilter=on  TunerSelectOption=Transfer Function Based (PID Tuner App)  InitialConditionSource=internal  InitialConditionForIntegrator=0  InitialConditionForFilter=0  DifferentiatorICPrevScaledInput=0  ExternalReset=none  TrackingMode=off  Kt=1  LimitOutput=on  SatLimitsSource=internal  UpperSaturationLimit=20  LowerSaturationLimit=-20  LinearizeAsGain=off  AntiWindupMode=clamping  Kb=1  LimitIntegrator=off  UpperIntegratorSaturationLimit=inf  LowerIntegratorSaturationLimit=-inf  POutMin=[]  POutMax=[]  IOutMin=[]  IOutMax=[]  DOutMin=[]  DOutMax=[]  NOutMin=[]  NOutMax=[]  SumOutMin=[]  SumOutMax=[]  SaturationOutMin=[]  SaturationOutMax=[]  PParamMin=[]  PParamMax=[]  IParamMin=[]  IParamMax=[]  DParamMin=[]  DParamMax=[]  NParamMin=[]  NParamMax=[]  KbParamMin=[]  KbParamMax=[]  KtParamMin=[]  KtParamMax=[]  KbOutMin=[]  KbOutMax=[]  KtOutMin=[]  KtOutMax=[]  IntegratorOutMin=[]  IntegratorOutMax=[]  FilterOutMin=[]  FilterOutMax=[]  SumI1OutMin=[]  SumI1OutMax=[]  SumI2OutMin=[]  SumI2OutMax=[]  SumI3OutMin=[]  SumI3OutMax=[]  SumI4OutMin=[]  SumI4OutMax=[]  SumDOutMin=[]  SumDOutMax=[]  DifferentiatorOutMin=[]  DifferentiatorOutMax=[]  FilterDiffOutCoefMin=[]  FilterDiffOutCoefMax=[]  ReciprocalOutMin=[]  ReciprocalOutMax=[]  SumDenOutMin=[]  SumDenOutMax=[]  SumNumOutMin=[]  SumNumOutMax=[]  DivideOutMin=[]  DivideOutMax=[]  UdiffTsProdOutMin=[]  UdiffTsProdOutMax=[]  NTsProdOutMin=[]  NTsProdOutMax=[]  UintegralTsProdOutMin=[]  UintegralTsProdOutMax=[]  UngainTsProdOutMin=[]  UngainTsProdOutMax=[]  ClampingZeroOutDataTypeStr=Inherit: Inherit via back propagation  ClampingZeroOutMin=[]  ClampingZeroOutMax=[]  FilterDenConstantOutDataTypeStr=Inherit: Inherit via back propagation  FilterDenConstantOutMin=[]  FilterDenConstantOutMax=[]  PCopyOutDataTypeStr=Inherit: Inherit via back propagation  PCopyOutMin=[]  PCopyOutMax=[]  NCopyOutDataTypeStr=Inherit: Inherit via back propagation  NCopyOutMin=[]  NCopyOutMax=[]  IntegratorContinuousStateAttributes=''  IntegratorStateMustResolveToSignalObject=off  IntegratorRTWStateStorageClass=Auto  FilterContinuousStateAttributes=''  FilterStateMustResolveToSignalObject=off  FilterRTWStateStorageClass=Auto  ParallelPVariant=InternalParameters  IdealPVariant=Disabled  IVariant=InternalParameters  DVariant=InternalParameters  IntegratorVariant=Continuous  SatVariant=Enabled  AWVariant=ContClampingParallel  PCopyVariant=Disabled  TRVariant=Disabled  FdbkBlocksVariant=Forward  IdealPFdbkVariant=Disabled  SatFdbkVariant=Disabled  DerivativeFilterVariant=ContFilter  NVariant=InternalParameters  NCopyVariant=Disabled  FilterICVariant=InternalICsFilter  IntegratorICVariant=InternalICs  ExternalResetVariant=Disabled  TRSumVariant=Passthrough  SumFdbkVariant=Disabled  SumVariant=Sum_PID  TsampFilterVariant=InternalTs  TsampNgainVariant=Passthrough  TsampIntegralVariant=Disabled_SignalSpec  ExternalSaturationOutDataTypeStr=Inherit: Same as second input
  Selector2 : Selector  InputPortWidth=3  IndexOptions=Index vector (dialog)  Indices=[1 2]  OutputSizes=1
  Selector4 : Selector  InputPortWidth=3  IndexOptions=Index vector (dialog)  Indices=[1 2]  OutputSizes=1
  Selector5 : Selector  InputPortWidth=3  IndexOptions=Index vector (dialog)  Indices=[3]  OutputSizes=1
  Selector6 : Selector  InputPortWidth=3  IndexOptions=Index vector (dialog)  Indices=[3]  OutputSizes=1
  Subtract3 : Sum  Inputs=|+-
  Subtract4 : Sum  Inputs=|+-
  Subtract5 : Sum  Inputs=|+-
  Terminator : Terminator
  Terminator1 : Terminator
  velocity reference : Scope
  vx_des : Outport
  vz_des : Outport  Port=2
  des_roll : Outport  Port=3
  wires:
  Gain/1 -> des_roll/1
  Selector6/1 -> Add2/2  "z"
  Mux/1 -> velocity reference/1
  Demux5/1 -> Subtract4/2  "x"
  PID_x1/1 -> Mux1/1, vx_des/1, Mux/1  "vx_cmd"
  Subtract4/1 -> PID_x1/1  "x_error"
  Demux6/1 -> Subtract3/2  "[vx vy]"
  Subtract3/1 -> Demux7/1
  Add2/1 -> PID_Altitude1/1  "z_error"
  PID_y1/1 -> Mux/2, Mux1/2  "vy_cmd"
  Reference_Pos/1 -> Selector5/1, Selector4/1
  Demux4/1 -> Subtract4/1  "x_cmd"
  PID_Altitude1/1 -> Mux/3, vz_des/1  "vz_cmd"
  Demux5/2 -> Subtract5/2  "y"
  Selector2/1 -> Demux5/1
  Current_Pos/1 -> Selector2/1, Selector6/1
  Demux4/2 -> Subtract5/1  "y_cmd"
  Subtract5/1 -> PID_y1/1  "y_error"
  Selector5/1 -> Add2/1
  Mux1/1 -> Subtract3/1
  Selector4/1 -> Demux4/1
  PID_vy1/1 -> Gain/1  "roll_cmd"
  Current_Vel/1 -> Demux6/1
  Demux7/2 -> PID_vy1/1  "vy_error"
  Demux6/2 -> Terminator/1  "vz"
  Demux7/1 -> Terminator1/1  "vx_error"

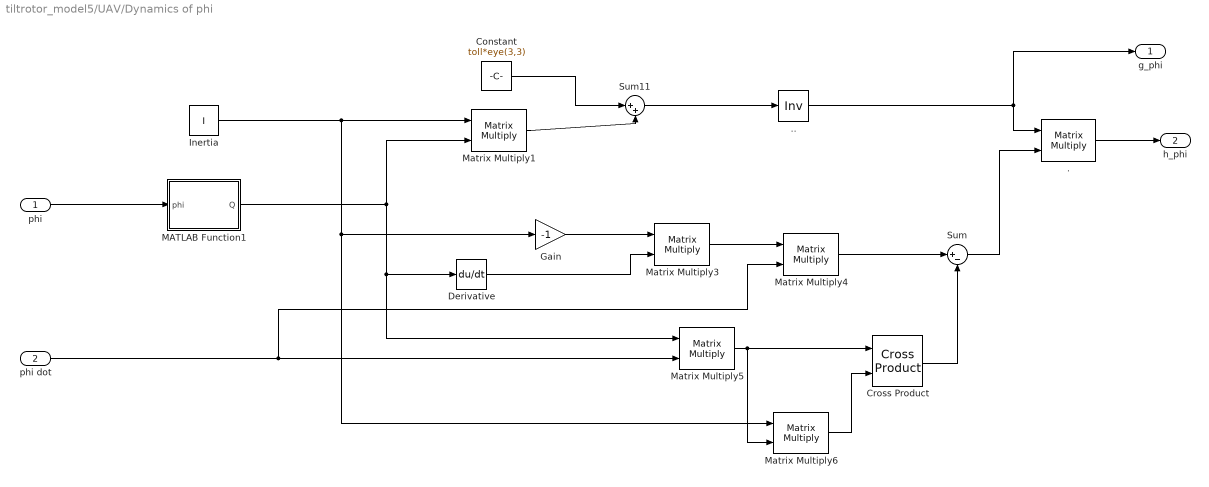
== system tiltrotor_model5/UAV/Dynamics of phi ==
  phi : Inport
  phi dot : Inport  Port=2
  . : Product  Multiplication=Matrix(*)
  .. : Product  Inputs=/  Multiplication=Matrix(*)
  Constant : Constant  Value=toll*eye(3,3)
  Cross Product : matrix_library/Cross Product
  Derivative : Derivative
  Gain : Gain  Gain=-1
  Inertia : Constant  Value=I  VectorParams1D=off
  MATLAB Function1 : MATLAB Function  TreatAsAtomicUnit=on
  Matrix Multiply{1,3..6} (5 alike) : Product  Multiplication=Matrix(*)
  Sum : Sum  Inputs=|+-
  Sum11 : Sum  Inputs=|++
  g_phi : Outport
  h_phi : Outport  Port=2
  wires:
  Matrix Multiply5/1 -> Matrix Multiply6/2, Cross Product/1
  Matrix Multiply4/1 -> Sum/1
  Gain/1 -> Matrix Multiply3/1
  ../1 -> ./1, g_phi/1
  Inertia/1 -> Matrix Multiply1/1, Matrix Multiply6/1, Gain/1
  Matrix Multiply3/1 -> Matrix Multiply4/1
  Cross Product/1 -> Sum/2
  Constant/1 -> Sum11/1
  Derivative/1 -> Matrix Multiply3/2
  MATLAB Function1/1(Q) -> Matrix Multiply5/1, Derivative/1, Matrix Multiply1/2
  Matrix Multiply6/1 -> Cross Product/2
  Sum/1 -> ./2
  Sum11/1 -> ../1
  phi dot/1 -> Matrix Multiply4/2, Matrix Multiply5/2
  Matrix Multiply1/1 -> Sum11/2
  phi/1 -> MATLAB Function1/1(phi)
  ./1 -> h_phi/1

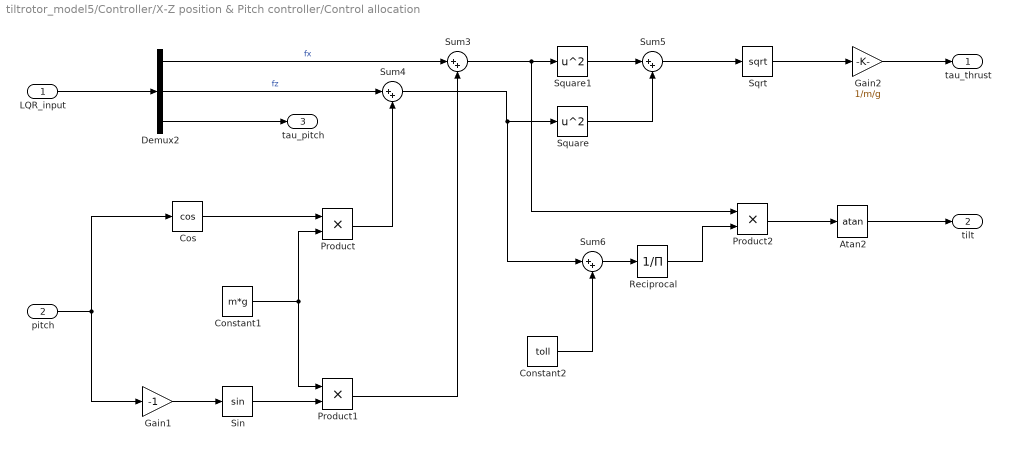
== system tiltrotor_model5/Controller/X-Z position & Pitch controller/Control allocation ==
  LQR_input : Inport
  pitch : Inport  Port=2
  Atan2 : Trigonometry  Operator=atan
  Constant1 : Constant  Value=m*g
  Constant2 : Constant  Value=toll
  Cos : Trigonometry  Operator=cos
  Demux2 : Demux  Outputs=3
  Gain1 : Gain  Gain=-1
  Gain2 : Gain  Gain=1/m/g
  Product : Product
  Product1 : Product
  Product2 : Product
  Reciprocal : Product  Inputs=/
  Sin : Trigonometry
  Sqrt : Sqrt
  Square : Math  Operator=square
  Square1 : Math  Operator=square
  Sum{3..6} (4 alike) : Sum  Inputs=|++
  tau_thrust : Outport
  tilt : Outport  Port=2
  tau_pitch : Outport  Port=3
  wires:
  Square1/1 -> Sum5/1
  pitch/1 -> Gain1/1, Cos/1
  Atan2/1 -> tilt/1
  Product1/1 -> Sum3/2
  Sin/1 -> Product1/2
  Sum6/1 -> Reciprocal/1
  Sum5/1 -> Sqrt/1
  Sqrt/1 -> Gain2/1
  Gain2/1 -> tau_thrust/1
  Product/1 -> Sum4/2
  Square/1 -> Sum5/2
  Cos/1 -> Product/1
  Sum3/1 -> Product2/1, Square1/1
  Constant2/1 -> Sum6/2
  Demux2/1 -> Sum3/1  "fx"
  Demux2/2 -> Sum4/1  "fz"
  Gain1/1 -> Sin/1
  Constant1/1 -> Product/2, Product1/1
  Reciprocal/1 -> Product2/2
  Sum4/1 -> Sum6/1, Square/1
  Demux2/3 -> tau_pitch/1
  LQR_input/1 -> Demux2/1
  Product2/1 -> Atan2/1
